simulink model "sysgenConv5x5"  (Simulink 7.2)
settings: Solver=ode45  StartTime=0.0  StopTime=64*64+2*64+30  RelTol=1e-3
PreLoadFcn:
  | sysgenConv5x5_PreLoadFcn
StopFcn:
  | sysgenConv5x5_StopFcn
libraries: xbsIndex_r4 x6, xrbsImage_r4 x2, xbsCopyrightNotice_r4 x1
settings Model: Creator=alexc  LastModifiedBy=juttu
settings DataIOCC: SignalLoggingName=sigsOut
settings OptimizationCC: BooleanDataType=off  InlineInvariantSignals=on  InitFltsAndDblsToZero=on
settings DebuggingCC: SaveWithParameterizedLinksMsg=none  SignalResolutionControl=TryResolveAllWithWarning  SolverPrmCheckMsg=none  MultiTaskDSMMsg=warning  MultiTaskCondExecSysMsg=none  StrictBusMsg=None
settings HardwareCC: TargetUnknown=on
settings RTWCC: IncludeERTFirstTime=on
settings GRTTargetCC: TargetFcnLib=ansi_tfl_tmw.mat

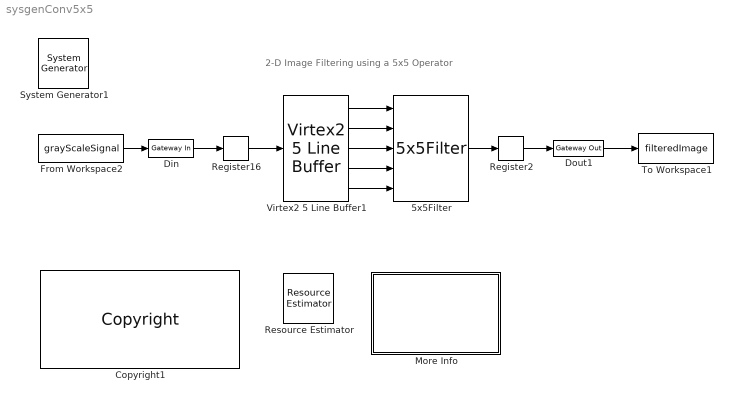
== system sysgenConv5x5 ==
  note: 2-D Image Filtering using a 5x5 Operator
  " System Generator1" : xbsIndex_r4/ System Generator  Tag=genX  SystemSampleTime=-1  xilinxfamily=virtex5  part=xc5vsx50t  speed=-1  package=ff1136  synthesis_tool=XST  clock_wrapper=Clock Enables  directory=./netlist  testbench=off  simulink_period=1/5  sysclk_period=4  dcm_input_clock_period=100  incr_netlist=off  trim_vbits=Everywhere in SubSystem  dbl_ovrd=According to Block Masks  core_generation=According to Block Masks  run_coregen=off  deprecated_control=off  eval_field=0  block_type=sysgen
      settings: block_version=9.2-dev
  5x5Filter : xrbsImage_r4/5x5Filter  SystemSampleTime=-1  maskNum=Edge  coef_n_bits=6  coef_bin_pt=0  smpl_n_bits=8  smpl_bin_pt=0  smpl_period=1  maskVal=0  maskDiv=0
      link override CMult: const=maskDiv(maskNum)  const_n_bits=18  const_bin_pt=17  en=off  latency=4  precision=Full  arith_type=Unsigned  n_bits=8  bin_pt=0  quantization=Truncate  overflow=Wrap  dbl_ovrd=off  use_behavioral_HDL=off  mem_type=Distributed RAM  pipeline=off  use_rpm=off  placement_style=Rectangular Shape
      link override CMult: xl_area=[0, 0, 0, 0, 0, 0, 0]
  Copyright1 : xbsCopyrightNotice_r4/Copyright  copyrighttext="Copyright (c) 2009  by  Xilinx, Inc. All rights reserved.<br><br>This file contains proprietary, confidential information of Xilinx, Inc., is distributed under licensefrom Xilinx, Inc., and may be used, copied and/or disclosed only pursuant to the terms of a valid licenseagreement with Xilinx, Inc. Xilinx hereby grants you a license to use this file solely for design,simulation, implementation and creation of design files limited to Xilinx devices or technologies. Use with non-Xilinx devices or technologies is expressly prohibited and immediately terminates your license unless covered by a separate agreement.<br><br>Xilinx is providing this design, code, or information \"as-is\" solely for use in developing programs and solutions for Xilinx devices, with no obligation on the part of Xilinx to provide support. By providingthis design, code, or information as one possible implementation of this feature, application or standard,Xilinx is making no representation that this implementation is free from any claims of infringement. Youare responsible for obtaining any rights you may require for your implementation. Xilinx expressly disclaimsany warranty whatsoever with respect to the adequacy of the implementation, including but not limited to anywarranties or representations that this implementation is free from claims of infringement, implied warrantiesof merchantability or fitness for a particular purpose.<br><br>Xilinx products are not intended for use in life support appliances, devices, or systems. Use in such applications is expressly prohibited.<br><br>Any modifications that are made to the Source Code are done at the user's sole risk and will be unsupported.<br><br>This copyright and support notice must be retained as part of this text at all times. (c) Copyright 1995-2009 Xilinx, Inc. All rights reserved."  block_type=copyright
      settings: block_version=10.1.00
      settings: infoedit=|
      | Copyright(C) 2008 by  Xilinx, Inc. All rights reserved.<br>
      | <br>
      | This file contains proprietary, confidential information of Xilinx, Inc., is distributed under license
      | from Xilinx, Inc., and may be used, copied and/or disclosed only pursuant to the terms of a valid license
      | agreement with Xilinx, Inc. Xilinx hereby grants you a license to use this file solely for design,
      | simulation, implementation and creation of design files limited to Xilinx devices or technologies. Use
      | with non-Xilinx devices or technologies is expressly prohibited and immediately terminates your license
      | unless covered by a separate agreement.<br>
      | <br>
      | Xilinx is providing this design, code, or information "as-is" solely for use in developing programs and
      | solutions for Xilinx devices, with no obligation on the part of Xilinx to provide support. By providing
      | this design, code, or information as one possible implementation of this feature, application or standard,
      | Xilinx is making no representation that this implementation is free from any claims of infringement. You
      | are responsible for obtaining any rights you may require for your implementation. Xilinx expressly disclaims
      | any warranty whatsoever with respect to the adequacy of the implementation, including but not limited to any
      | warranties or representations that this implementation is free from claims of infringement, implied warranties
      | of merchantability or fitness for a particular purpose.<br>
      | <br>
      | Xilinx products are not intended for use in life support appliances, devices, or systems. Use in such
      | applications is expressly prohibited.<br>
      | <br>
      | Any modifications that are made to the Source Code are done at the user's sole risk and will be unsupported.<br>
      | <br>
      | This copyright and support notice must be retained as part of this text at all times.
      | (c) Copyright 1995-2008 Xilinx, Inc. All rights reserved.
  Din : xbsIndex_r4/Gateway In  arith_type=Unsigned  n_bits=8  bin_pt=0  quantization="Round  (unbiased: +/- Inf)"  overflow=Saturate  period=1  dbl_ovrd=off  timing_constraint=None  locs_specified=off  LOCs={}  block_type=gatewayin
      settings: infoedit="Gateway in block.  Converts inputs of type Simulink integer, double and fixed point to  Xilinx fixed point type.<P><P>Hardware notes:  In hardware these blocks become top level input ports."  xl_area=[0 0 0 0 8 0 0]  block_version=VER_STRING_GOES_HERE
  Dout1 : xbsIndex_r4/Gateway Out  hdl_port=on  timing_constraint="Data Rate;  Set 'FAST' Attribute"  locs_specified=off  LOCs={}  block_type=gatewayout
      settings: infoedit="Gateway out block.  Converts Xilinx fixed point inputs into ouputs of type Simulink integer, double, or fixed point.<P><P>Hardware notes:  In hardware these blocks become top level output ports or are discarded, depending on how they are configured."  xl_area=[0 0 0 0 8 0 0]  block_version=VER_STRING_GOES_HERE
  From Workspace2 : FromWorkspace  VariableName=grayScaleSignal  SampleTime=1  Interpolate=off  OutputAfterFinalValue=Setting to zero
  More Info : Subsystem
      mask Display: disp('Double click\n for\n more information.')
  Register16 : xbsIndex_r4/Register  init=0  rst=off  en=off  dbl_ovrd=off  block_type=register
      settings: xl_area=[4 8 0 0 0 0 0]  block_version=VER_STRING_GOES_HERE
  Register2 : xbsIndex_r4/Register  init=0  rst=off  en=off  dbl_ovrd=off  block_type=register
      settings: xl_area=[4 8 0 0 0 0 0]  block_version=VER_STRING_GOES_HERE
  Resource Estimator : xbsIndex_r4/Resource Estimator  Tag=resEstTag  Slices=353  FFs=573  BRAMs=9  LUTs=377  IOBs=16  EBMs=5  TBUFs=0  xl_use_estimator_area=off  est_options=Estimate  xl_estimator_area=[353 573 9 377 16 5 0]  mrp_directory=./sysgenConv5x5_work  simulink_period=1/5  block_type=resource_estimator
      settings: AttributesFormatString=Resource\nEstimator  block_version=9.2-dev
  To Workspace1 : ToWorkspace  VariableName=filteredImage  SampleTime=1  SaveFormat=Array
  Virtex2 5 Line Buffer1 : xrbsImage_r4/Virtex2 5 Line Buffer  SystemSampleTime=-1  line_size=64  cst=1
  wires:
  Din/1 -> Register16/1
  From Workspace2/1 -> Din/1
  Register16/1 -> Virtex2 5 Line Buffer1/1
  Dout1/1 -> To Workspace1/1
  Register2/1 -> Dout1/1
  5x5Filter/1 -> Register2/1
  Virtex2 5 Line Buffer1/1 -> 5x5Filter/1
  Virtex2 5 Line Buffer1/2 -> 5x5Filter/2
  Virtex2 5 Line Buffer1/3 -> 5x5Filter/3
  Virtex2 5 Line Buffer1/4 -> 5x5Filter/4
  Virtex2 5 Line Buffer1/5 -> 5x5Filter/5

== system sysgenConv5x5/More Info ==
  note: This design shows how a 2-D Image filter can be realized efficiently using
      | n-tap MAC FIR Filters.  The filters used in the '5x5 Filter' subsystem are from
      | the Custom FIR library provided as a System Generator demo.
      |
      | This demo is configured to process 64x64 grayscale image. Nine different 2-D
      | filters have been provided.  The filter can be selected by changing  the mask
      | parameter on the 5x5 Filter block   The 2-D filter coefficients are stored in a block
      | RAM, and the model makes no specific optimizations for these coefficients.
      | You can substitute your own coefficients by modifying the mask of the 5x5 filter
      | block, under the Initialization tab.
      |
      | This design occupies 340 Slice LUTs, 536 Slice Registers,
      | 5 dedicated multipliers, and 5 Block RAMs of a Xilinx xc5vs50t-1 part and operates
      | at  250MHz (10.1.3 software, VHDL synthesized with XST).
      |
      | The underlying 5-tap MAC FIR filters are clocked 5 times faster than the input rate.
      | Therefore the throughput of the design is 250 MHz / 5 = 50 million pixels/ second.
      | For a 64x64 image, this is 50x10^6/(64x64) = 12,207 frames/sec.  For a 256x256
      | image the throughput would be 763 frames /sec, and for a 512x512 image it would
      | be  190 frames/sec.
  note: 2-D Image Filtering using a 5x5 Operator
